simulink model "vehicles"  (R2020a)
settings: Solver=VariableStepAuto  StartTime=0.0  StopTime=10.0  RelTol=1e-3
undefined symbols (not defined in the file or in its folder): L, ld, psi_o1, psi_o10, psi_o2, psi_o3, psi_o4, psi_o5, psi_o6, psi_o7, psi_o8, psi_o9, X_last1, X_last10, X_last2, X_last3, X_last4, X_last5, X_last6, X_last7, X_last8, X_last9, X_o, X_o1, X_o10, X_o2, X_o3, X_o4, X_o5, X_o6, X_o7, X_o8, X_o9, xRef1, xRef10, xRef2, xRef3, xRef4, xRef5, xRef6, xRef7, xRef8, xRef9, Y_last1, Y_last10, Y_last2, Y_last3, Y_last4, Y_last5, Y_last6, Y_last7, Y_last8, Y_last9, Y_o, Y_o1, Y_o10, Y_o2, Y_o3, Y_o4, Y_o5 ... (+14)
libraries: autolibutils x40, autolibshared x30, robotalgslib x10, simulink x10, vdynlib x10
(part 15 of 18)

== system vehicles/vehicle 7/Powertrain & Driveline1/Powertrain ==
  Acc : Inport
  AxlPwr : Inport  Port=2
  Omega : Inport  Port=3
  Abs : Abs  ZeroCross=off
  Constant3 : Constant  Value=0
  Diff Torque : Gain  Gain=1000
  Divide : Product  Inputs=*/
  EngPwr : Constant  Value=100e3
  Gear : Constant  SampleTime=-1
  Max : MinMax  Function=max  ZeroCross=off
  Powertrain : autolibutils/Cont LPF  wc=4*pi*2  aMode=2
      settings: SourceProductBaseCode=PW,MT,AR,VE,VP
  Saturation : Saturate  UpperLimit=inf  LowerLimit=0  ZeroCross=off
  Saturation Dynamic1 : simulink/Discontinuities/Saturation Dynamic  OutMin=[]  OutMax=[]  OutDataTypeStr=Inherit: Same as second input  OutDataType=fixdt(1, 16)  OutScaling=2^-10  DoSatur=off
  Saturation2 : Saturate  UpperLimit=inf  LowerLimit=100  ZeroCross=off
  Saturation3 : Saturate  UpperLimit=1000  LowerLimit=0  ZeroCross=off
  Subtract : Sum  Inputs=+-
  Sum of Elements : Sum  Inputs=+
  Switch : Switch  ZeroCross=off
  Tip Out : Gain  Gain=-10
  div0protect : autolibutils/div0protect - poly  thresh=1  aMode=2
      settings: SourceProductBaseCode=PW,MT,AR,VE,VP
  AxlTrq : Outport  VectorParamsAs1DForOutWhenUnconnected=off
  wires:
  Max/1 -> div0protect/1
  Saturation3/1 -> Saturation Dynamic1/1  "AxlTrqLim"
  AxlPwr/1 -> Sum of Elements/1
  EngPwr/1 -> Subtract/1
  Saturation2/1 -> Divide/1  "PwrLim"
  Subtract/1 -> Saturation2/1
  Omega/1 -> Max/1
  div0protect/1 -> Divide/2
  Divide/1 -> Saturation3/1
  Abs/1 -> Subtract/2
  Sum of Elements/1 -> Abs/1
  Constant3/1 -> Saturation Dynamic1/3
  Tip Out/1 -> Switch/3
  Saturation Dynamic1/1 -> Powertrain/1
  Gear/1 -> Switch/2
  Diff Torque/1 -> Saturation Dynamic1/2
  Saturation/1 -> Diff Torque/1
  Acc/1 -> Switch/1, Tip Out/1
  Switch/1 -> Saturation/1
  Powertrain/1 -> AxlTrq/1

== system vehicles/vehicle 8/Lateral and Longitudinal Controller1/Pure Pursuit Controller ==
  note: The subsystem implements a Pure Pursuit controller. The "Pure Pursuit" block calculates the target direction and the "Wheel Steering Angle Formulation" block calculates the wheel steering angle.
  Pose : Inport
  Waypoints : Inport  Port=2
  Pure Pursuit : robotalgslib/Pure Pursuit  DesiredLinearVelocity=0.5  MaxAngularVelocity=1.0  LookaheadDistance=ld  TargetDirPort=on  SimulateUsing=Code generation
  Terminator6 : Terminator
  Terminator7 : Terminator
  Wheel Steering Angle Formulation : Subsystem  mask{L=L, ld=ld}
      mask prompts: L "Bicycle length"; ld "Lookahead distance"
      mask TypeOptions L: Bicycle length/Value
      mask TypeOptions ld: Lookahead distance/Value
      mask Display:
      | image("GeometryMask.png")
      | port_label('input', 1, 'alpha')
      | port_label('output', 1, 'delta')
  delta : Outport
  AngularVelocity : Outport  Port=2
  wires:
  Pure Pursuit/1 -> Terminator6/1
  Pose/1 -> Pure Pursuit/1
  Pure Pursuit/2 -> Terminator7/1, AngularVelocity/1
  Waypoints/1 -> Pure Pursuit/2
  Pure Pursuit/3 -> Wheel Steering Angle Formulation/1(alpha)
  Wheel Steering Angle Formulation/1(Al) -> delta/1

== system vehicles/vehicle 8/Lateral and Longitudinal Controller1/Stop-system ==
  acel : Inport
  xCar : Inport  Port=2
  decel : Inport  Port=3
  yCar : Inport  Port=4
  Abs{1..6} (6 alike) : Abs
  Add1 : Sum  Inputs=-+
  Add2 : Sum  Inputs=-+
  Constant1 : Constant  Value=3
  Constant2 : Constant  Value=0
  Constant3 : Constant
  Constant4 : Constant  Value=X_last8
  Constant5 : Constant  Value=Y_last8
  Logical Operator : Logic  AllPortsSameDT=off  OutDataTypeStr=boolean
  Relational Operator : RelationalOperator  Operator=<=  OutDataTypeStr=boolean  RndMeth=Simplest
  Relational Operator1 : RelationalOperator  Operator=<=  OutDataTypeStr=boolean  RndMeth=Simplest
  Switch : Switch  Criteria=u2 > Threshold
  Switch1 : Switch  Criteria=u2 > Threshold
  AcelCmd : Outport
  DecelCmd : Outport  Port=2
  wires:
  Abs1/1 -> Add2/1
  xCar/1 -> Abs4/1
  Logical Operator/1 -> Switch/2, Switch1/2
  acel/1 -> Switch/3
  Abs5/1 -> Relational Operator1/1
  Relational Operator1/1 -> Logical Operator/2
  Abs6/1 -> Relational Operator/1
  Abs3/1 -> Add1/2
  Switch/1 -> AcelCmd/1
  Add1/1 -> Abs6/1
  Constant2/1 -> Switch/1
  Constant5/1 -> Abs2/1
  yCar/1 -> Abs1/1
  Abs4/1 -> Add1/1
  Relational Operator/1 -> Logical Operator/1
  Constant3/1 -> Switch1/1
  Constant4/1 -> Abs3/1
  Abs2/1 -> Add2/2
  Switch1/1 -> DecelCmd/1
  Constant1/1 -> Relational Operator1/2, Relational Operator/2
  decel/1 -> Switch1/3
  Add2/1 -> Abs5/1

== system vehicles/vehicle 8/Powertrain & Driveline1/Brake System ==
  Decc : Inport
  Hydraulics : autolibutils/Cont LPF  wc=30*pi*2  aMode=2
      settings: SourceProductBaseCode=PW,MT,AR,VE,VP
  Pressure : Gain  Gain=2e7
  Saturation1 : Saturate  UpperLimit=inf  LowerLimit=0  ZeroCross=off
  Selector : Selector  InputPortWidth=1  IndexOptions=Index vector (dialog)  Indices=[1 1 1 1]  OutputSizes=1
  Signal Specification : SignalSpecification  Unit=Pa
  Prs : Outport  VectorParamsAs1DForOutWhenUnconnected=off
  wires:
  Pressure/1 -> Selector/1
  Hydraulics/1 -> Pressure/1
  Saturation1/1 -> Hydraulics/1
  Selector/1 -> Signal Specification/1
  Decc/1 -> Saturation1/1
  Signal Specification/1 -> Prs/1
